simulink model "DBX_model_all"  (R2015a)
settings: Solver=ode2  SolverMode=SingleTasking  StartTime=0.0  StopTime=10.0  FixedStep=T_sim  RelTol=1e-3
values from neighbouring files (symbols this model uses):
  A_M = 2/sqrt(3)*L_M    [SetupComplete.m]    (also in simple_all.m = single(A_M))
  Alpha_unique_rad = deg2rad(Alpha_unique)    [DBX_aero_V1.m]    (also in simple_all.m = single(Alpha_unique_rad))
  as = aerosonde_data_mod    [SetupComplete.m]
  B_span = 3    [SetupComplete.m]    (also in simple_all.m = single(B_span))
  Beta_unique_rad = deg2rad(Beta_unique)    [DBX_aero_V1.m]    (also in simple_all.m = single(Beta_unique_rad))
  C_D_q = 0.0336    [DBX_aero_V1.m]    (also in simple_all.m = single(C_D_q))
  C_l = NaN*ones(size(Alpha_unique,1),size(Beta_unique,1) )    [DBX_aero_V1.m]    (also in simple_all.m = single(C_l))
  C_l_delta_a_Asim = C_l_raw(idx)/deg2rad(delta_ale(idx))    [DBX_aero_V1.m]    (also in simple_all.m = single(C_l_delta_a_Asim))
  C_l_delta_rv_Asim = C_l_raw(idx)/deg2rad(delta_rud(idx))    [DBX_aero_V1.m]    (also in simple_all.m = single(C_l_delta_rv_Asim))
  C_l_p = -0.8333    [DBX_aero_V1.m]    (also in simple_all.m = single(C_l_p))
  C_l_r = 0.0347    [DBX_aero_V1.m]    (also in simple_all.m = single(C_l_r))
  C_Lift_q = 10.9    [DBX_aero_V1.m]    (also in simple_all.m = single(C_Lift_q))
  C_m = NaN*ones(size(Alpha_unique,1),size(Beta_unique,1),size(delta_elev_unique,1) )    [DBX_aero_V1.m]    (also in simple_all.m = single(C_m))
  C_m_q = -45.7828    [DBX_aero_V1.m]    (also in simple_all.m = single(C_m_q))
  C_n = NaN*ones(size(Alpha_unique,1),size(Beta_unique,1) )    [DBX_aero_V1.m]    (also in simple_all.m = single(C_n))
  C_n_delta_a_Asim = C_n_raw(idx)/deg2rad(delta_ale(idx))    [DBX_aero_V1.m]    (also in simple_all.m = single(C_n_delta_a_Asim))
  C_n_delta_rv_Asim = C_n_raw(idx)/deg2rad(delta_rud(idx))    [DBX_aero_V1.m]    (also in simple_all.m = single(C_n_delta_rv_Asim))
  C_n_p = -0.0066    [DBX_aero_V1.m]    (also in simple_all.m = single(C_n_p))
  C_n_r = -0.1827    [DBX_aero_V1.m]    (also in simple_all.m = single(C_n_r))
  C_X = NaN*ones(size(Alpha_unique,1),size(Beta_unique,1),size(delta_elev_unique,1) )    [DBX_aero_V1.m]    (also in simple_all.m = single(C_X))
  C_Y = NaN*ones(size(Alpha_unique,1),size(Beta_unique,1) )    [DBX_aero_V1.m]    (also in simple_all.m = single(C_Y))
  C_Y_delta_rv_Asim = C_y(idx)/deg2rad(delta_rud(idx))    [DBX_aero_V1.m]    (also in simple_all.m = single(C_Y_delta_rv_Asim))
  C_Y_p = -0.0991    [DBX_aero_V1.m]    (also in simple_all.m = single(C_Y_p))
  C_Y_r = 0.5219    [DBX_aero_V1.m]    (also in simple_all.m = single(C_Y_r))
  C_Z = NaN*ones(size(Alpha_unique,1),size(Beta_unique,1),size(delta_elev_unique,1) )    [DBX_aero_V1.m]    (also in simple_all.m = single(C_Z))
  CG = (m_OE*CG_OE + m_PL*CG_PL)/m    [SetupComplete.m]    (also in simple_all.m = single(CG))
  CMA = 0.25    [SetupComplete.m]    (also in simple_all.m = single(CMA))
  delta_elev_unique_rad = deg2rad(delta_elev_unique)    [DBX_aero_V1.m]    (also in simple_all.m = single(delta_elev_unique_rad))
  g = 9.81    [SetupComplete.m]    (also in simple_all.m = single(g))
  h_1 = -0.0666    [SetupComplete.m]    (also in simple_all.m = single(h_1))
  h_2 = -0.0666    [SetupComplete.m]    (also in simple_all.m = single(h_2))
  h_3 = -0.04824    [SetupComplete.m]    (also in simple_all.m = single(h_3))
  I_BAC = I_CG + m*[CG(3)^2,0,CG(1)*CG(3);0,CG(1)^2+CG(3)^2,0;CG(1)*CG(3),0,CG(1)^2]    [SetupComplete.m]    (also in simple_all.m = single(I_BAC))
  Initial_Omegas = max(0,Omega_0)    [Run_DBX.m]    (also in simple_all.m = single(Initial_Omegas))
  Initial_Torques = Torque_0    [Run_DBX.m]    (also in simple_all.m = single(Initial_Torques))
  L_M = 1.20    (= 1.2)    [SetupComplete.m]    (also in simple_all.m = single(L_M))
  m = m_OE + m_PL    (= 14.5)    [SetupComplete.m]    (also in simple_all.m = single(m))
  Rotation_sign = [-1,-1,-1]    [SetupComplete.m]    (also in simple_all.m = single(Rotation_sign))
undefined symbols (not defined in the file or in its folder): DOWN_0, EAST_0, F, MIL, NORTH_0, P_0, Q_0, R_0, Servo_calib, U_0, V_0, W_0
libraries: DBX_model x14, aerolibwind2 x6, aerolibasang x5, aerolibadyn x2, aerolibtransform2 x1
(part 2 of 2)

== system DBX_model_all/aeromodel/Aero model/Aerodynamics/Force Coefficients/C_Z_T ==
  note: Deflexiones efectivas:
      |
      | delta_ail_Asim
      | delta_rv_sim
      | delta_rv_Asim
  alpha : Inport
  beta : Inport  Port=2
  body_rates_adim : Inport  Port=3  PortDimensions=[3 1]
  defl_control : Inport  Port=4
  Add : Sum  Inputs=++|
  Add1 : Sum  Inputs=--|
  C_D_q : Constant  Value=C_D_q
  C_Lift_q : Constant  Value=C_Lift_q
  C_Z : Lookup_n-D  NumberOfTableDimensions=3  BreakpointsForDimension1=Alpha_unique_rad  BreakpointsForDimension2=Beta_unique_rad  BreakpointsForDimension3=delta_elev_unique_rad  Table=C_Z  DiagnosticForOutOfRangeInput=Warning  RemoveProtectionInput=on  InternalRulePriority=Speed  RndMeth=Simplest  InputSameDT=on
  Divide : Product  Inputs=**
  Divide1 : Product  Inputs=**
  Divide2 : Product  Inputs=**
  Selector : Selector  InputPortWidth=3  Indices=2
  Selector1 : Selector  InputPortWidth=3  Indices=2
  cos : Trigonometry  Operator=cos
  sin : Trigonometry
  C_Z_T : Outport
  wires:
  Add/1 -> C_Z_T/1
  Divide/1 -> Add/2
  C_Z/1 -> Add/1
  Selector/1 -> Divide/1
  body_rates_adim/1 -> Selector/1
  beta/1 -> C_Z/2
  alpha/1 -> cos/1, sin/1, C_Z/1
  defl_control/1 -> Selector1/1
  Selector1/1 -> C_Z/3
  cos/1 -> Divide1/1
  C_Lift_q/1 -> Divide1/2
  C_D_q/1 -> Divide2/2
  Divide1/1 -> Add1/2
  Divide2/1 -> Add1/1
  sin/1 -> Divide2/1
  Add1/1 -> Divide/2

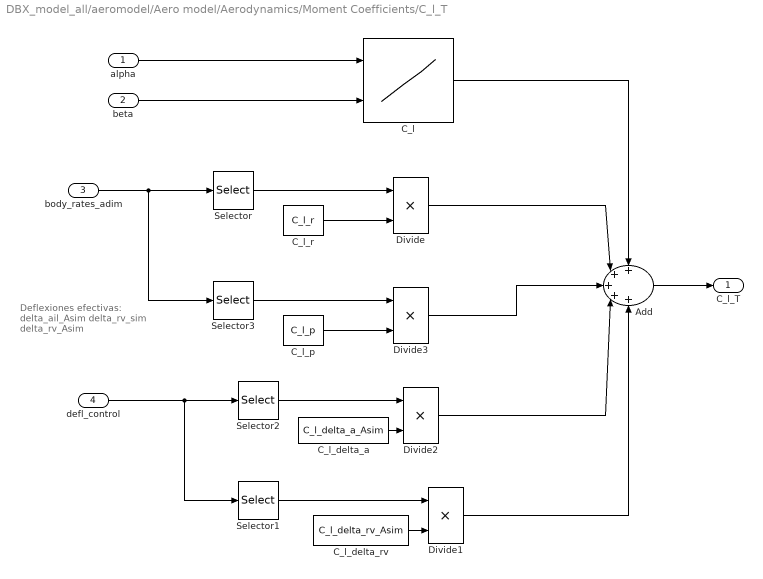
== system DBX_model_all/aeromodel/Aero model/Aerodynamics/Moment Coefficients/C_l_T ==
  note: Deflexiones efectivas:
      |
      | delta_ail_Asim
      | delta_rv_sim
      | delta_rv_Asim
  alpha : Inport
  beta : Inport  Port=2
  body_rates_adim : Inport  Port=3  PortDimensions=[3 1]
  defl_control : Inport  Port=4
  Add : Sum  Inputs=+++++
  C_l : Lookup_n-D  BreakpointsForDimension1=Alpha_unique_rad  BreakpointsForDimension2=Beta_unique_rad  Table=C_l  DiagnosticForOutOfRangeInput=Warning  RemoveProtectionInput=on  InternalRulePriority=Speed  RndMeth=Simplest  InputSameDT=on
  C_l_delta_a : Constant  Value=C_l_delta_a_Asim
  C_l_delta_rv : Constant  Value=C_l_delta_rv_Asim
  C_l_p : Constant  Value=C_l_p
  C_l_r : Constant  Value=C_l_r
  Divide{,1..3} (4 alike) : Product  Inputs=**
  Selector : Selector  InputPortWidth=3  Indices=3
  Selector1 : Selector  InputPortWidth=3  Indices=3
  Selector2 : Selector  InputPortWidth=3
  Selector3 : Selector  InputPortWidth=3
  C_l_T : Outport
  wires:
  alpha/1 -> C_l/1
  beta/1 -> C_l/2
  Add/1 -> C_l_T/1
  defl_control/1 -> Selector1/1, Selector2/1
  C_l_delta_a/1 -> Divide2/2
  Selector2/1 -> Divide2/1
  C_l_delta_rv/1 -> Divide1/2
  Selector1/1 -> Divide1/1
  C_l_r/1 -> Divide/2
  body_rates_adim/1 -> Selector3/1, Selector/1
  Selector3/1 -> Divide3/1
  C_l_p/1 -> Divide3/2
  Selector/1 -> Divide/1
  C_l/1 -> Add/1
  Divide/1 -> Add/2
  Divide3/1 -> Add/3
  Divide2/1 -> Add/4
  Divide1/1 -> Add/5

== system DBX_model_all/aeromodel/Aero model/Aerodynamics/Moment Coefficients/C_m_T ==
  note: Deflexiones efectivas:
      |
      | delta_ail_Asim
      | delta_rv_sim
      | delta_rv_Asim
  alpha : Inport
  beta : Inport  Port=2
  body_rates_adim : Inport  Port=3  PortDimensions=[3 1]
  defl_control : Inport  Port=4
  Add : Sum  Inputs=++|
  C_m : Lookup_n-D  NumberOfTableDimensions=3  BreakpointsForDimension1=Alpha_unique_rad  BreakpointsForDimension2=Beta_unique_rad  BreakpointsForDimension3=delta_elev_unique_rad  Table=C_m  DiagnosticForOutOfRangeInput=Warning  RemoveProtectionInput=on  InternalRulePriority=Speed  RndMeth=Simplest  InputSameDT=on
  C_m_q : Constant  Value=C_m_q
  Divide : Product  Inputs=**
  Selector : Selector  InputPortWidth=3  Indices=2
  Selector2 : Selector  InputPortWidth=3  Indices=2
  C_m_T : Outport
  wires:
  alpha/1 -> C_m/1
  Selector/1 -> Divide/1
  C_m_q/1 -> Divide/2
  body_rates_adim/1 -> Selector/1
  defl_control/1 -> Selector2/1
  Divide/1 -> Add/2
  C_m/1 -> Add/1
  Add/1 -> C_m_T/1
  Selector2/1 -> C_m/3
  beta/1 -> C_m/2

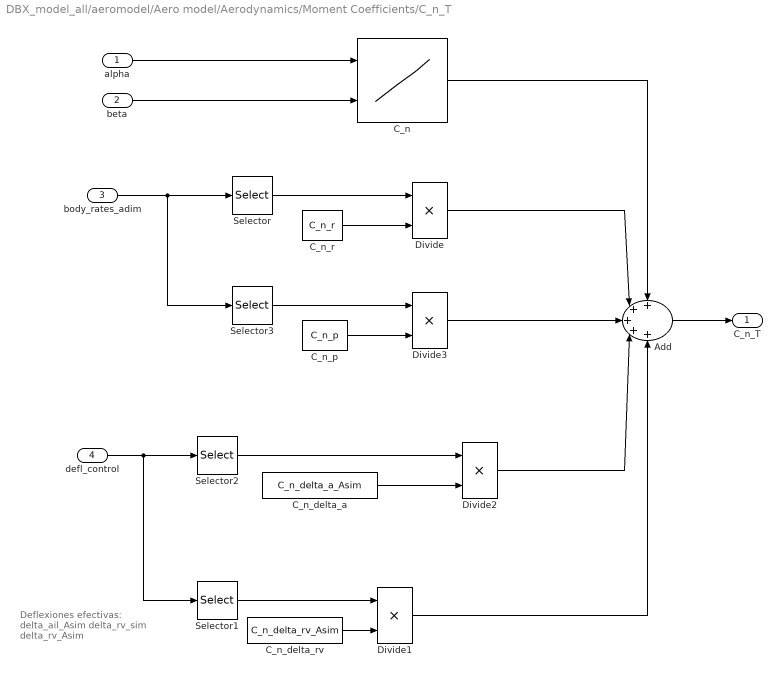
== system DBX_model_all/aeromodel/Aero model/Aerodynamics/Moment Coefficients/C_n_T ==
  note: Deflexiones efectivas:
      |
      | delta_ail_Asim
      | delta_rv_sim
      | delta_rv_Asim
  alpha : Inport
  beta : Inport  Port=2
  body_rates_adim : Inport  Port=3  PortDimensions=[3 1]
  defl_control : Inport  Port=4
  Add : Sum  Inputs=+++++
  C_n : Lookup_n-D  BreakpointsForDimension1=Alpha_unique_rad  BreakpointsForDimension2=Beta_unique_rad  Table=C_n  DiagnosticForOutOfRangeInput=Warning  RemoveProtectionInput=on  InternalRulePriority=Speed  RndMeth=Simplest  InputSameDT=on
  C_n_delta_a : Constant  Value=C_n_delta_a_Asim
  C_n_delta_rv : Constant  Value=C_n_delta_rv_Asim
  C_n_p : Constant  Value=C_n_p
  C_n_r : Constant  Value=C_n_r
  Divide{,1..3} (4 alike) : Product  Inputs=**
  Selector : Selector  InputPortWidth=3  Indices=3
  Selector1 : Selector  InputPortWidth=3  Indices=3
  Selector2 : Selector  InputPortWidth=3
  Selector3 : Selector  InputPortWidth=3
  C_n_T : Outport
  wires:
  alpha/1 -> C_n/1
  beta/1 -> C_n/2
  Add/1 -> C_n_T/1
  defl_control/1 -> Selector1/1, Selector2/1
  C_n_delta_a/1 -> Divide2/2
  Selector2/1 -> Divide2/1
  C_n_delta_rv/1 -> Divide1/2
  Selector1/1 -> Divide1/1
  C_n_r/1 -> Divide/2
  body_rates_adim/1 -> Selector3/1, Selector/1
  Selector3/1 -> Divide3/1
  C_n_p/1 -> Divide3/2
  Selector/1 -> Divide/1
  C_n/1 -> Add/1
  Divide/1 -> Add/2
  Divide3/1 -> Add/3
  Divide2/1 -> Add/4
  Divide1/1 -> Add/5

== system DBX_model_all/aeromodel/Aero model/Aerodynamics/Wind-axes Velocities/Calculate alphadot ==
  note: Calculate alphadot
  note: W
  "[Udot Vdot Wdot]" : Inport
  "[U V W]" : Inport  Port=2
  Demux : Demux  Outputs=3
  Demux1 : Demux  Outputs=3
  Math Function : Math  Operator=square  SaturateOnIntegerOverflow=on
  Math Function1 : Math  Operator=square  SaturateOnIntegerOverflow=on
  Product : Product  RndMeth=Zero
  Product1 : Product  RndMeth=Zero
  Product2 : Product  Inputs=*/  RndMeth=Zero
  Sum : Sum  Inputs=-|+
  Sum1 : Sum  Inputs=+|+
  Terminator : Terminator
  Terminator1 : Terminator
  alphadot : Outport
  wires:
  Product2/1 -> alphadot/1  "alphadot"
  "[Udot Vdot Wdot]"/1 -> Demux/1
  "[U V W]"/1 -> Demux1/1
  Demux1/2 -> Terminator1/1
  Sum/1 -> Product2/1
  Product/1 -> Sum/2  "U Wdot"
  Product1/1 -> Sum/1  "W Udot"
  Sum1/1 -> Product2/2  "U^2 + W^2"
  Math Function1/1 -> Sum1/2
  Math Function/1 -> Sum1/1
  Demux1/3 -> Math Function1/1, Product1/2
  Demux1/1 -> Math Function/1, Product/2  "U"
  Demux/2 -> Terminator/1
  Demux/3 -> Product/1  "Wdot"
  Demux/1 -> Product1/1  "Udot"

== system DBX_model_all/aeromodel/Aero model aerosonde/Aerodynamics/Force Coefficients/Drag Coefficients ==
  note: Drag coefficient
  control : Inport
  Mach : Inport  Port=2
  CL : Inport  Port=3  PortDimensions=1
  (CL-CL0)^2/(pi e AR) : Gain  Gain=1/as.pieaR  Multiplication=Matrix(K*u)  SaturateOnIntegerOverflow=on  OutDataTypeStr=Inherit: Same as input  ParamDataTypeStr=Inherit: Same as input
  Abs4 : Abs  SaturateOnIntegerOverflow=on
  CDM : Gain  Gain=as.CDM  SaturateOnIntegerOverflow=on  OutDataTypeStr=Inherit: Same as input  ParamDataTypeStr=Inherit: Same as input
  CDdf : Gain  Gain=[as.CDdf, as.CDde, as.CDda, as.CDdr]  Multiplication=Matrix(K*u)  SaturateOnIntegerOverflow=on  OutDataTypeStr=Inherit: Same as input  ParamDataTypeStr=Inherit: Same as input
  CL min drag : Constant  Value=as.CLmind
  CL^2 : Math  Operator=square  SaturateOnIntegerOverflow=on
  Constant terms : Constant  Value=as.CD0
  Sum : Sum  Inputs=|+-  SaturateOnIntegerOverflow=on  InputSameDT=on  OutDataTypeStr=Inherit: Same as first input
  Sum1 : Sum  Inputs=++++  SaturateOnIntegerOverflow=on  InputSameDT=on  OutDataTypeStr=Inherit: Same as first input
  CD : Outport
  wires:
  (CL-CL0)^2/(pi e AR)/1 -> Sum1/4
  CL min drag/1 -> Sum/2
  CL/1 -> Sum/1
  Sum/1 -> CL^2/1
  CL^2/1 -> (CL-CL0)^2/(pi e AR)/1
  Sum1/1 -> CD/1  "CD"
  Mach/1 -> CDM/1
  control/1 -> Abs4/1
  Abs4/1 -> CDdf/1
  CDM/1 -> Sum1/3
  CDdf/1 -> Sum1/2
  Constant terms/1 -> Sum1/1

== system DBX_model_all/aeromodel/Aero model aerosonde/Aerodynamics/Force Coefficients/Lift Coefficients ==
  note: Lift Coefficients
  alpha : Inport
  control : Inport  Port=2
  alphadot : Inport  Port=3
  pqr : Inport  Port=4
  2V_a : Inport  Port=5
  Mach : Inport  Port=6
  CL*c/(2V_a) : Product  Inputs=*/  SaturateOnIntegerOverflow=on  InputSameDT=on  OutDataTypeStr=Inherit: Same as first input
  CL0 : Constant  Value=as.CL0
  CLM : Gain  Gain=as.CLM  SaturateOnIntegerOverflow=on  OutDataTypeStr=Inherit: Same as input  ParamDataTypeStr=Inherit: Same as input
  CLalpha : Gain  Gain=as.CLalpha  SaturateOnIntegerOverflow=on  OutDataTypeStr=Inherit: Same as input  ParamDataTypeStr=Inherit: Same as input
  CLalphadot : Gain  Gain=as.CLalphadot  Multiplication=Matrix(K*u)  SaturateOnIntegerOverflow=on  OutDataTypeStr=Inherit: Same as input  ParamDataTypeStr=Inherit: Same as input
  CLq : Gain  Gain=[0, as.CLq, 0]  Multiplication=Matrix(K*u)  SaturateOnIntegerOverflow=on  OutDataTypeStr=Inherit: Same as input  ParamDataTypeStr=Inherit: Same as input
  Sum : Sum  SaturateOnIntegerOverflow=on  InputSameDT=on  OutDataTypeStr=Inherit: Same as first input
  Sum2 : Sum  Inputs=+++++  SaturateOnIntegerOverflow=on  InputSameDT=on  OutDataTypeStr=Inherit: Same as first input
  "[CLdf, CLde, 0, 0]" : Gain  Gain=[as.CLdf, as.CLde, 0, 0]  Multiplication=Matrix(K*u)  SaturateOnIntegerOverflow=on  OutDataTypeStr=Inherit: Same as input  ParamDataTypeStr=Inherit: Same as input
  c : Gain  Gain=as.c  SaturateOnIntegerOverflow=on  OutDataTypeStr=Inherit: Same as input  ParamDataTypeStr=Inherit: Same as input
  CL : Outport
  wires:
  alphadot/1 -> CLalphadot/1
  alpha/1 -> CLalpha/1
  Mach/1 -> CLM/1
  2V_a/1 -> CL*c/(2V_a)/2
  pqr/1 -> CLq/1
  control/1 -> "[CLdf, CLde, 0, 0]"/1
  c/1 -> CL*c/(2V_a)/1
  CL*c/(2V_a)/1 -> Sum2/4
  CLM/1 -> Sum2/5
  Sum2/1 -> CL/1  "CL"
  "[CLdf, CLde, 0, 0]"/1 -> Sum2/3
  CLalpha/1 -> Sum2/2
  CL0/1 -> Sum2/1
  Sum/1 -> c/1
  CLalphadot/1 -> Sum/1
  CLq/1 -> Sum/2

== system DBX_model_all/aeromodel/Aero model aerosonde/Aerodynamics/Force Coefficients/Side Force Coefficients ==
  note: Side force coefficients
  beta : Inport
  control : Inport  Port=2
  angular rates : Inport  Port=3
  2V_a : Inport  Port=4
  CY*b/(2V_a) : Product  Inputs=*/  SaturateOnIntegerOverflow=on  InputSameDT=on  OutDataTypeStr=Inherit: Same as first input
  CYbeta : Gain  Gain=as.CYbeta  SaturateOnIntegerOverflow=on  OutDataTypeStr=Inherit: Same as input  ParamDataTypeStr=Inherit: Same as input
  Sum3 : Sum  Inputs=+++  SaturateOnIntegerOverflow=on  InputSameDT=on  OutDataTypeStr=Inherit: Same as first input
  Wing span1 : Gain  Gain=as.b  SaturateOnIntegerOverflow=on  OutDataTypeStr=Inherit: Same as input  ParamDataTypeStr=Inherit: Same as input
  "[0, 0, CYda, CYdr]" : Gain  Gain=[0, 0, as.CYda, as.CYdr]  Multiplication=Matrix(K*u)  SaturateOnIntegerOverflow=on  OutDataTypeStr=Inherit: Same as input  ParamDataTypeStr=Inherit: Same as input
  "[CYp, 0, CYr]" : Gain  Gain=[as.CYp, 0, as.CYr]  Multiplication=Matrix(K*u)  SaturateOnIntegerOverflow=on  OutDataTypeStr=Inherit: Same as input  ParamDataTypeStr=Inherit: Same as input
  CY : Outport
  wires:
  beta/1 -> CYbeta/1
  2V_a/1 -> CY*b/(2V_a)/2
  angular rates/1 -> "[CYp, 0, CYr]"/1
  control/1 -> "[0, 0, CYda, CYdr]"/1
  Wing span1/1 -> CY*b/(2V_a)/1
  Sum3/1 -> CY/1  "CY"
  CY*b/(2V_a)/1 -> Sum3/3
  "[0, 0, CYda, CYdr]"/1 -> Sum3/2
  CYbeta/1 -> Sum3/1
  "[CYp, 0, CYr]"/1 -> Wing span1/1

== system DBX_model_all/aeromodel/Aero model aerosonde/Aerodynamics/Moment Coefficients/Pitch Moment Coefficients ==
  alpha : Inport
  control : Inport  Port=2
  alphadot : Inport  Port=3
  pqr : Inport  Port=4
  2V_a : Inport  Port=5
  Mach : Inport  Port=6
  CMalpha : Gain  Gain=as.Cmalpha  SaturateOnIntegerOverflow=on  OutDataTypeStr=Inherit: Same as input  ParamDataTypeStr=Inherit: Same as input
  Cm*c/(2V_a) : Product  Inputs=*/  SaturateOnIntegerOverflow=on  InputSameDT=on  OutDataTypeStr=Inherit: Same as first input
  Cm0 : Constant  Value=as.Cm0
  CmM : Gain  Gain=as.CmM  SaturateOnIntegerOverflow=on  OutDataTypeStr=Inherit: Same as input  ParamDataTypeStr=Inherit: Same as input
  Cmalphadot : Gain  Gain=as.Cmalphadot  Multiplication=Matrix(K*u)  SaturateOnIntegerOverflow=on  OutDataTypeStr=Inherit: Same as input  ParamDataTypeStr=Inherit: Same as input
  Cmq : Gain  Gain=[0, as.Cmq, 0]  Multiplication=Matrix(K*u)  SaturateOnIntegerOverflow=on  OutDataTypeStr=Inherit: Same as input  ParamDataTypeStr=Inherit: Same as input
  Sum : Sum  SaturateOnIntegerOverflow=on  InputSameDT=on  OutDataTypeStr=Inherit: Same as first input
  Sum2 : Sum  Inputs=+++++  SaturateOnIntegerOverflow=on  InputSameDT=on  OutDataTypeStr=Inherit: Same as first input
  "[Cmdf, Cmde, 0, 0]" : Gain  Gain=[as.Cmdf, as.Cmde, 0, 0]  Multiplication=Matrix(K*u)  SaturateOnIntegerOverflow=on  OutDataTypeStr=Inherit: Same as input  ParamDataTypeStr=Inherit: Same as input
  c : Gain  Gain=as.c  SaturateOnIntegerOverflow=on  OutDataTypeStr=Inherit: Same as input  ParamDataTypeStr=Inherit: Same as input
  Cm : Outport
  wires:
  Cmq/1 -> Sum/2
  Cmalphadot/1 -> Sum/1
  Sum/1 -> c/1
  Cm0/1 -> Sum2/1
  CMalpha/1 -> Sum2/2
  "[Cmdf, Cmde, 0, 0]"/1 -> Sum2/3
  Sum2/1 -> Cm/1  "Cm"
  CmM/1 -> Sum2/5
  Cm*c/(2V_a)/1 -> Sum2/4
  c/1 -> Cm*c/(2V_a)/1
  control/1 -> "[Cmdf, Cmde, 0, 0]"/1
  pqr/1 -> Cmq/1
  2V_a/1 -> Cm*c/(2V_a)/2
  Mach/1 -> CmM/1
  alpha/1 -> CMalpha/1
  alphadot/1 -> Cmalphadot/1

== system DBX_model_all/aeromodel/Aero model aerosonde/Aerodynamics/Moment Coefficients/Roll Moment Coefficients ==
  note: Roll moment coefficient
  beta : Inport
  control : Inport  Port=2
  angular rates : Inport  Port=3
  2V : Inport  Port=4
  CY*b/(2V) : Product  Inputs=*/  SaturateOnIntegerOverflow=on  InputSameDT=on  OutDataTypeStr=Inherit: Same as first input
  Clbeta : Gain  Gain=as.Clbeta  SaturateOnIntegerOverflow=on  OutDataTypeStr=Inherit: Same as input  ParamDataTypeStr=Inherit: Same as input
  Sum3 : Sum  Inputs=+++  SaturateOnIntegerOverflow=on  InputSameDT=on  OutDataTypeStr=Inherit: Same as first input
  Wing span : Gain  Gain=as.b  SaturateOnIntegerOverflow=on  OutDataTypeStr=Inherit: Same as input  ParamDataTypeStr=Inherit: Same as input
  "[0, 0, Clda, Cldr]" : Gain  Gain=[0, 0, as.Clda, as.Cldr]  Multiplication=Matrix(K*u)  SaturateOnIntegerOverflow=on  OutDataTypeStr=Inherit: Same as input  ParamDataTypeStr=Inherit: Same as input
  "[Clp, 0, Clr]" : Gain  Gain=[as.Clp, 0, as.Clr]  Multiplication=Matrix(K*u)  SaturateOnIntegerOverflow=on  OutDataTypeStr=Inherit: Same as input  ParamDataTypeStr=Inherit: Same as input
  Cl : Outport
  wires:
  "[Clp, 0, Clr]"/1 -> Wing span/1
  Clbeta/1 -> Sum3/1
  "[0, 0, Clda, Cldr]"/1 -> Sum3/2
  CY*b/(2V)/1 -> Sum3/3
  Sum3/1 -> Cl/1  "Cl"
  Wing span/1 -> CY*b/(2V)/1
  control/1 -> "[0, 0, Clda, Cldr]"/1
  angular rates/1 -> "[Clp, 0, Clr]"/1
  2V/1 -> CY*b/(2V)/2
  beta/1 -> Clbeta/1

== system DBX_model_all/aeromodel/Aero model aerosonde/Aerodynamics/Moment Coefficients/Yaw Moment Coefficients ==
  note: Yaw moment coefficient
  beta : Inport
  control : Inport  Port=2
  angular rates : Inport  Port=3
  2V_a : Inport  Port=4
  Cn*b/(2V_a) : Product  Inputs=*/  SaturateOnIntegerOverflow=on  InputSameDT=on  OutDataTypeStr=Inherit: Same as first input
  Cnbeta : Gain  Gain=as.Cnbeta  SaturateOnIntegerOverflow=on  OutDataTypeStr=Inherit: Same as input  ParamDataTypeStr=Inherit: Same as input
  Sum3 : Sum  Inputs=+++  SaturateOnIntegerOverflow=on  InputSameDT=on  OutDataTypeStr=Inherit: Same as first input
  Wing span : Gain  Gain=as.b  SaturateOnIntegerOverflow=on  OutDataTypeStr=Inherit: Same as input  ParamDataTypeStr=Inherit: Same as input
  "[0, 0, Cnda, Cndr]" : Gain  Gain=[0, 0, as.Cnda, as.Cndr]  Multiplication=Matrix(K*u)  SaturateOnIntegerOverflow=on  OutDataTypeStr=Inherit: Same as input  ParamDataTypeStr=Inherit: Same as input
  "[Cnp, 0, Cnr]" : Gain  Gain=[as.Cnp, 0, as.Cnr]  Multiplication=Matrix(K*u)  SaturateOnIntegerOverflow=on  OutDataTypeStr=Inherit: Same as input  ParamDataTypeStr=Inherit: Same as input
  Cn : Outport
  wires:
  beta/1 -> Cnbeta/1
  2V_a/1 -> Cn*b/(2V_a)/2
  angular rates/1 -> "[Cnp, 0, Cnr]"/1
  control/1 -> "[0, 0, Cnda, Cndr]"/1
  Wing span/1 -> Cn*b/(2V_a)/1
  Sum3/1 -> Cn/1  "Cn"
  Cn*b/(2V_a)/1 -> Sum3/3
  "[0, 0, Cnda, Cndr]"/1 -> Sum3/2
  Cnbeta/1 -> Sum3/1
  "[Cnp, 0, Cnr]"/1 -> Wing span/1

== system DBX_model_all/aeromodel/Aero model aerosonde/Aerodynamics/Wind-axes Velocities/Calculate alphadot ==
  note: Calculate alphadot
  note: W
  "[Udot Vdot Wdot]" : Inport
  "[U V W]" : Inport  Port=2
  Demux : Demux  Outputs=3
  Demux1 : Demux  Outputs=3
  Math Function : Math  Operator=square  SaturateOnIntegerOverflow=on
  Math Function1 : Math  Operator=square  SaturateOnIntegerOverflow=on
  Product : Product  RndMeth=Zero
  Product1 : Product  RndMeth=Zero
  Product2 : Product  Inputs=*/  RndMeth=Zero
  Sum : Sum  Inputs=-|+
  Sum1 : Sum  Inputs=+|+
  Terminator : Terminator
  Terminator1 : Terminator
  alphadot : Outport
  wires:
  Product2/1 -> alphadot/1  "alphadot"
  "[Udot Vdot Wdot]"/1 -> Demux/1
  "[U V W]"/1 -> Demux1/1
  Demux1/2 -> Terminator1/1
  Sum/1 -> Product2/1
  Product/1 -> Sum/2  "U Wdot"
  Product1/1 -> Sum/1  "W Udot"
  Sum1/1 -> Product2/2  "U^2 + W^2"
  Math Function1/1 -> Sum1/2
  Math Function/1 -> Sum1/1
  Demux1/3 -> Math Function1/1, Product1/2
  Demux1/1 -> Math Function/1, Product/2  "U"
  Demux/2 -> Terminator/1
  Demux/3 -> Product/1  "Wdot"
  Demux/1 -> Product1/1  "Udot"

== matlab function DBX_model_all/6dof Eqs of motion/Position Eqs ==
  data: A_b output; Vb input; omega input; omega_dot input; Forces input; m input; CG input
function A_b  = PositionEqs(Vb,omega,omega_dot, Forces,m, CG)



 
A_b =  1/m*( Forces ) - cross(omega,Vb) - cross(omega, cross(omega,CG)) -cross(omega_dot,CG)  ;

== matlab function DBX_model_all/6dof Eqs of motion/Rotational eqs ==
  data: omega_dot output; omega_b input; Moments input; I_BAC input
function omega_dot  = Rotational_Eq(omega_b,Moments, I_BAC)



omega_dot =  I_BAC\( Moments - cross(omega_b,I_BAC*omega_b)  );

== matlab function DBX_model_all/6dof Eqs of motion/q_dot/Quaternion_dot ==
  data: omega_b input; q_dot output; q input
function q_dot = Quaternion_dot(omega_b,q)


q_dot = 1/2*HamiltonProduct(q,[0;omega_b]);

== matlab function DBX_model_all/aeromodel/Aero model aerosonde/ISA ==
  data: altitude input; rho output; T output; Ps output; a output
function [rho,T,Ps,a]= ISA_atmos(altitude)


    rho0 = 1.225; tfac = 1 - 6.5e-3/288.15*altitude;
    T = 288.15*tfac; if (altitude >= 11000) T = 216.65; end;
    rho = rho0*(tfac.^4.2586);
    Ps = 287*rho*T;
    a=sqrt(1.4*287*T);
    
end

== matlab function DBX_model_all/aeromodel/Aero model/ISA ==
  data: altitude input; rho output; T output; Ps output; a output
function [rho,T,Ps,a]= ISA_atmos(altitude)


    rho0 = 1.225; tfac = 1 - 6.5e-3/288.15*altitude;
    T = 288.15*tfac; if (altitude >= 11000) T = 216.65; end;
    rho = rho0*(tfac.^4.2586);
    Ps = 287*rho*T;
    a=sqrt(1.4*287*T);
    
end

== matlab function DBX_model_all/6dof Eqs of motion/Eccelerometer meas ==
  data: Vb input; omega input; omega_dot input; Ab input; A_s output; r_sens parameter
function A_s  = AcellMeas(Vb,omega,omega_dot,Ab, r_sens)




A_s =  Ab + cross(omega,Vb) + cross(omega, cross(omega,r_sens)) +cross(omega_dot,r_sens)  ;

== matlab function DBX_model_all/6dof Eqs of motion/SVFI_to_SVFb ==
  data: X_e input; V_e input; X_e_out output; V_b output; omega_b output; Euler_Ang input; Euler_Ang_Dot input; q output
function [X_e_out,V_b, omega_b ,q]=SVFI_to_SVFb(X_e,V_e, Euler_Ang,Euler_Ang_Dot)

q = zeros(4,1);
V_b =zeros(3,1);

xp=V_e(1);
yp=V_e(2);
zp=V_e(3);

phi=Euler_Ang(1);
theta=Euler_Ang(2);
psi=Euler_Ang(3);
phip=Euler_Ang_Dot(1);
thetap=Euler_Ang_Dot(2);
psip=Euler_Ang_Dot(3);

%%
X_e_out=X_e;

q = QuaternionfromEuler(phi,theta,psi); 



HamOut=HamiltonProduct([q(1);-q(2);-q(3);-q(4)],HamiltonProduct([0;xp;yp;zp],[q(1);q(2);q(3);q(4)]) );% q* . v . q
V_b=HamOut(2:4);

omega_b=[phip-psip*sin(theta)  ;
         thetap*cos(phi)+psip*cos(theta)*sin(phi);
            -thetap*sin(phi)+psip*cos(theta)*cos(phi)  ];% Ya que es solo una operacion aislada utilizaremos la ecuaciones con rel trigonometricas

function [q]=QuaternionfromEuler(phi,theta,psi)
% options=optimset('MaxFunEvals',3000);
% q=fsolve(@QUATERNIONEULER,[0.6,0.4,0.5,0.4]); % Hay que acertar con los angulos poniendo diferentes valores iniciales del quaternion
%     function F=QUATERNIONEULER(q)
%         F=[ tan(phi)-(2*q(3)*q(4)-2*q(1)*q(2))/(2*q(1)^2+2*q(4)^2-1)  ;
%             sin(-theta)-2*q(2)*q(4)-2*q(1)*q(3);
%             tan(psi)-(2*q(2)*q(3)-2*q(1)*q(4))/(2*q(1)^2+2*q(2)^2-1);
%             q(1)^2+q(2)^2+q(3)^2+q(4)^2-1];
%     end  % Este algoritmo da q* !!!!!

q=[ cos(psi/2)*cos(theta/2)*cos(phi/2)+ sin(psi/2)*sin(theta/2)*sin(phi/2) ;
      cos(psi/2)*cos(theta/2)*sin(phi/2)- sin(psi/2)*sin(theta/2)*cos(phi/2) ;
       cos(psi/2)*sin(theta/2)*cos(phi/2)+ sin(psi/2)*cos(theta/2)*sin(phi/2)   ;
        sin(psi/2)*cos(theta/2)*cos(phi/2)- cos(psi/2)*sin(theta/2)*sin(phi/2)      ]; % Esto nos da q !!!

    function Product= HamiltonProduct( a,b )

Product=[ a(1)*b(1)-a(2)*b(2)-a(3)*b(3)-a(4)*b(4) ; a(1)*b(2)+a(2)*b(1)+a(3)*b(4)-a(4)*b(3)  ; a(1)*b(3)-a(2)*b(4)+a(3)*b(1)+a(4)*b(2)  ; a(1)*b(4)+a(2)*b(3)-a(3)*b(2)+a(4)*b(1) ];

== matlab function DBX_model_all/6dof Eqs of motion/SV_F_b_to_SV_FI ==
  data: V_b input; q_dot input; q input; V_e output; euler output; euler_dot output
function [V_e,euler,euler_dot]   = SV_F_b_to_SV_FI(  V_b, q_dot,q)

xp=V_b(1);
yp=V_b(2);
zp=V_b(3);

%% Velocity and position in Earth Frame   q . v . q*

SolProd=HamiltonProduct([q(1);q(2);q(3);q(4)],HamiltonProduct([0;xp;yp;zp],[q(1);-q(2);-q(3);-q(4)]) );
V_e=SolProd(2:4);

%% Actitud en Angulos de Euler y sus derivadas. 
euler=[0,0,0]';
euler(1,1) = atan2(2*q(3)*q(4)+2*q(1)*q(2),2*q(1)^2+2*q(4)^2-1 ); % phi
euler(2,1) = -asin( 2*q(2)*q(4)-2*q(1)*q(3) ); %  theta
euler(3,1) = atan2( 2*q(2)*q(3)+2*q(1)*q(4),2*q(1)^2+2*q(2)^2-1 ); %  psi

euler_dot=[0,0,0]';
euler_dot(1,1) = 2/(1+( (2*q(3)*q(4)+2*q(1)*q(2))/(2*q(1)^2+2*q(4)^2-1)  )^2)*[ -(2*q(1)^2*q(2)+ 4*q(1)*q(3)*q(4)-2*q(2)*q(4)^2+q(2))  ,  q(1)*(2*q(1)^2+2*q(4)^2-1)  ,  q(4)*(2*q(1)^2+2*q(4)^2-1)  ,  -(-2*q(1)^2*q(3) +4*q(1)*q(2)*q(4)+2*q(3)*q(4)^2+q(3) ) ]*q_dot.* 1/(2*q(1)^2+2*q(4)^2-1)^2; % Derivada de phi
euler_dot(2,1) = -2/( sqrt(1-4*(q(2)*q(4)-q(1)*q(3))^2)  )*[-q(3),q(4),-q(1),q(2)]*q_dot;  % Theta prima
euler_dot(3,1) = 2/(1+( (2*q(2)*q(3)+2*q(1)*q(4))/(2*q(1)^2+2*q(2)^2-1)  )^2)*[  -(2*q(1)^2*q(4)+4*q(1)*q(2)*q(3)-2*q(2)^2*q(4)+q(4)  ) , 1/2*(q(3)*(4*q(1)^2-4*q(2)^2-2)-8*q(1)*q(2)*q(4) )  ,  q(2)*(2*q(1)^2+2*q(2)^2-1)  , q(1)*(2*q(1)^2+2*q(2)^2-1) ]*q_dot.*1/(2*q(1)^2+2*q(2)^2-1)^2;  % Psi prima


function Product= HamiltonProduct( a,b )

Product=[ a(1)*b(1)-a(2)*b(2)-a(3)*b(3)-a(4)*b(4) ; a(1)*b(2)+a(2)*b(1)+a(3)*b(4)-a(4)*b(3)  ; a(1)*b(3)-a(2)*b(4)+a(3)*b(1)+a(4)*b(2)  ; a(1)*b(4)+a(2)*b(3)-a(3)*b(2)+a(4)*b(1) ];
